simulink model "KD_cl_harness_cl_ouports_added"  (R2015b)
settings: Solver=ode45  StartTime=0  StopTime=inf  FixedStep=0.01  MaxStep=0.005  RelTol=1e-5  AbsTol=1e-5
undefined symbols (not defined in the file or in its folder): A2, bin_vec, c_0, c_1000, c_1000inv, c_100inv, c_1d2p4, c_1p7, c_4400inv, c_5500inv, c_80, c_compmap, c_ctok, c_fflow_max, c_fflow_min, c_filt, c_flowdiv, c_flowmin, c_flowmult, c_inf, c_km1d2k, c_n1, c_p00001, c_p01, c_p1e9, c_p4d1p4, c_pincomp, c_rair, c_roacorr, c_rpmtoradpers, c_svrthrottle1, c_svrthrottle2, c_svrthrottlearg, c_svrthrottlebeta, c_vnliftmax, c_vnliftmin, cl_offset, clff, Coefs, const, const_exhat, const_vec, Dual_array, dual_zero, egr_ecu_ff, expcon, f_mat, gs_jul, HQP_eps, HQP_INF, HQP_saturation, IV, L2, length_L, maxL, mHQP_saturation, minL, Newton, nRed, num_constraints ... (+22)
libraries: simulink x33
(part 4 of 6)

== system KD_cl_harness_cl_ouports_added/ctrl_rb_explicit_20140220_v6_simp/scheduled_observer/observer ==
  map : Inport
  egrr : Inport  Port=2
  xhatROpm : Inport  Port=3
  u : Inport  Port=4  OutDataTypeStr=single
  Action Port : ActionPort  ActionType=then
  Gain : Gain  Gain=expcon.RobsC  Multiplication=Matrix(K*u) (u vector)
      settings: AttributesFormatString=%<Multiplication>
  Gain1 : Gain  Gain=expcon.RobsL  Multiplication=Matrix(K*u) (u vector)
      settings: AttributesFormatString=%<Multiplication>
  Gain2 : Gain  Gain=expcon.RobsA  Multiplication=Matrix(K*u) (u vector)
      settings: AttributesFormatString=%<Multiplication>
  Gain3 : Gain  Gain=expcon.RobsB  Multiplication=Matrix(K*u) (u vector)
      settings: AttributesFormatString=%<Multiplication>
  Gain4 : Gain  Gain=expcon.RobsD  Multiplication=Matrix(K*u) (u vector)
      settings: AttributesFormatString=%<Multiplication>
  Mux : Mux  Inputs=2
  Mux1 : Mux  Inputs=3
  Sum : Sum  Inputs=++|
  Sum1 : Sum  Inputs=|+-
  Sum2 : Sum  Inputs=|++
  Sum3 : Sum  Inputs=+-|
  Sum4 : Sum  Inputs=-+|
  Sum5 : Sum  Inputs=+-|
  Unit Delay{1..4,7..8} (6 alike) : UnitDelay  SampleTime=-1
      settings: AttributesFormatString=%<X0>
  xhatRO : Outport  OutDataTypeStr=single
  xhat : Outport  Port=2  InitialOutput=[0,0,0,0,0,0]
  wires:
  Sum5/1 -> Mux/2
  Unit Delay4/1 -> Sum5/2
  Sum3/1 -> Mux/1
  Unit Delay3/1 -> Sum3/2
  Unit Delay1/1 -> Mux1/2
  Unit Delay2/1 -> Mux1/3
  [map] -> Unit Delay1/1
  [egrr] -> Unit Delay2/1
  Mux1/1 -> xhat/1
  Gain/1 -> Sum1/2
  Sum4/1 -> Sum1/1
  Gain3/1 -> Sum2/2
  Sum/1 -> Sum2/1
  xhatROpm/1 -> Unit Delay7/1
  map/1 -> Sum3/1, Unit Delay3/1, [map]
  egrr/1 -> Sum5/1, Unit Delay4/1, [egrr]
  Sum1/1 -> Gain1/1
  Gain1/1 -> Sum/1
  Gain2/1 -> Sum/2
  u/1 -> Unit Delay8/1
  Mux/1 -> Sum4/2
  Gain4/1 -> Sum4/1
  Sum2/1 -> Mux1/1, xhatRO/1
  Unit Delay8/1 -> Gain3/1, Gain4/1
  Unit Delay7/1 -> Gain/1, Gain2/1

== system KD_cl_harness_cl_ouports_added/ctrl_rb_explicit_20140220_v6_simp/set_point_maps/EGR_rate_map ==
  fuel_rate_mm3perst : Inport
  engine_speed : Inport  Port=2
  egr_ecu : Lookup2D  RowIndex=egr_ecu_ff.x  ColumnIndex=egr_ecu_ff.y  Table=egr_ecu_ff.z  LookUpMeth=Interpolation-Use End Values
      settings: AttributesFormatString=%<LookUpMeth>\n%<RowIndex>\n%<ColumnIndex>\n%<Table>
  EGR_rate_ref : Outport
  wires:
  egr_ecu/1 -> EGR_rate_ref/1
  fuel_rate_mm3perst/1 -> egr_ecu/2
  engine_speed/1 -> egr_ecu/1

== system KD_cl_harness_cl_ouports_added/ctrl_rb_explicit_20140220_v6_simp/set_point_maps/intake_pressure_map ==
  fuel_rate_mm3perst : Inport
  engine_speed : Inport  Port=2
  boost_pressure_map : Subsystem
  intake_manifold_pressure_ref : Outport
  wires:
  engine_speed/1 -> boost_pressure_map/2(engine_speed)
  fuel_rate_mm3perst/1 -> boost_pressure_map/1(fuel_rate_mm3perst)
  boost_pressure_map/1(intake_manifold_pressure) -> intake_manifold_pressure_ref/1

== system KD_cl_harness_cl_ouports_added/pre-throttle manifold/p_preThrottle/Cus_integrator ==
  in : Inport
  p_prethrottle (kPa)1 : Integrator  InitialCondition=IV.p_prethrottle  UpperSaturationLimit=maxL.p_PreThrottle  LowerSaturationLimit=minL.p_PreThrottle
  p_preThrottle : Outport
  wires:
  p_prethrottle (kPa)1/1 -> p_preThrottle/1
  in/1 -> p_prethrottle (kPa)1/1

== system KD_cl_harness_cl_ouports_added/EGR Throttle/EGR Throttle/Throttle Model2/Air Model_map_use ==
  TA[deg] : Inport
  Ne[rpm] : Inport  Port=2
  Pim[Pa] : Inport  Port=3
  Tim[K] : Inport  Port=4
  Pa[Pa] : Inport  Port=5
  Ta[K] : Inport  Port=6
  R_im : Inport  Port=7
  R_a : Inport  Port=8
  Back-Flow : Subsystem
  Forward-Flow : Subsystem
  Gain : Gain  Gain=-1
  Product : Product  Inputs=/*  SaturateOnIntegerOverflow=on  RndMeth=Zero  InputSameDT=on  OutDataTypeStr=Inherit: Same as first input
  Product1 : Product  Inputs=*//  SaturateOnIntegerOverflow=on  RndMeth=Zero  InputSameDT=on  OutDataTypeStr=Inherit: Same as first input
  Product3 : Product  Inputs=*//  SaturateOnIntegerOverflow=on  RndMeth=Zero  InputSameDT=on  OutDataTypeStr=Inherit: Same as first input
  Switch : Switch  Threshold=1  SaturateOnIntegerOverflow=on  InputSameDT=on
  mt[kg/sec] : Outport
  forwardmt : Outport  Port=2
  backwardmt : Outport  Port=3
  sat_out-37 : Outport  Port=4
  sat_out-38 : Outport  Port=5
  sat_out-39 : Outport  Port=6
  sat_out-40 : Outport  Port=7
  out-1 : Outport  Port=8
  out-3 : Outport  Port=9
  out-4 : Outport  Port=10
  wires:
  Product1/1 -> Forward-Flow/1(Ro_a)
  Switch/1 -> mt[kg/sec]/1
  Product/1 -> Switch/2, out-1/1
  TA[deg]/1 -> Forward-Flow/2(TA[deg]), Back-Flow/1(TA[deg])
  [Pa] -> Product/2, Forward-Flow/4(Pa), Back-Flow/4(Pa)
  Pim[Pa]/1 -> Forward-Flow/5(Pm), Product/1, Back-Flow/5(Pm), Product3/1
  Pa[Pa]/1 -> [Pa]
  Ta[K]/1 -> [Ta]
  R_a/1 -> [Ra]
  R_im/1 -> [Rim]
  [Ra] -> Product1/3
  [Pa] -> Product1/1
  [Ta] -> Product1/2
  [Rim] -> Product3/3
  Tim[K]/1 -> Product3/2
  Forward-Flow/1(mt_dot[kg/s]) -> Switch/1, forwardmt/1
  Product3/1 -> Back-Flow/3(Ro_m)
  Back-Flow/1(mt_dot[kg/s]) -> Gain/1
  Ne[rpm]/1 -> Forward-Flow/3(Ne[rpm]), Back-Flow/2(Ne[rpm])
  Gain/1 -> Switch/3, backwardmt/1
  Back-Flow/2(sat_out-37) -> sat_out-37/1
  Back-Flow/3(sat_out-38) -> sat_out-38/1
  Forward-Flow/2(sat_out-39) -> sat_out-39/1
  Forward-Flow/3(sat_out-40) -> sat_out-40/1
  Back-Flow/4(out-3) -> out-3/1
  Forward-Flow/4(out-4) -> out-4/1

== system KD_cl_harness_cl_ouports_added/EGR Valve/SVR EGR/EGR_model/Air Model_map_use ==
  TA[deg] : Inport
  Ne[rpm] : Inport  Port=2
  Pim[Pa] : Inport  Port=3
  Tim[K] : Inport  Port=4
  Pa[Pa] : Inport  Port=5
  Ta[K] : Inport  Port=6
  R_im : Inport  Port=7
  R_a : Inport  Port=8
  Back-Flow : Subsystem
  Forward-Flow : Subsystem
  Gain : Gain  Gain=-1
  Product : Product  Inputs=/*  SaturateOnIntegerOverflow=on  RndMeth=Zero  InputSameDT=on  OutDataTypeStr=Inherit: Same as first input
  Product1 : Product  Inputs=*//  SaturateOnIntegerOverflow=on  RndMeth=Zero  InputSameDT=on  OutDataTypeStr=Inherit: Same as first input
  Product3 : Product  Inputs=*//  SaturateOnIntegerOverflow=on  RndMeth=Zero  InputSameDT=on  OutDataTypeStr=Inherit: Same as first input
  Switch : Switch  Threshold=1  SaturateOnIntegerOverflow=on  InputSameDT=on
  mt[kg/sec] : Outport
  forwardmt : Outport  Port=2
  sat_out-41 : Outport  Port=3
  sat_out-42 : Outport  Port=4
  sat_out-43 : Outport  Port=5
  sat_out-44 : Outport  Port=6
  out-2 : Outport  Port=7
  out-5 : Outport  Port=8
  out-6 : Outport  Port=9
  wires:
  Ne[rpm]/1 -> Back-Flow/2(Ne[rpm]), Forward-Flow/3(Ne[rpm])
  Back-Flow/1(mt_dot[kg/s]) -> Gain/1  "rv"
  Product3/1 -> Back-Flow/3(Ro_m)
  Forward-Flow/1(mt_dot[kg/s]) -> forwardmt/1, Switch/1  "ff"
  Tim[K]/1 -> Product3/2
  [Rim] -> Product3/3
  [Ta] -> Product1/2
  [Pa] -> Product1/1
  [Ra] -> Product1/3
  R_im/1 -> [Rim]
  R_a/1 -> [Ra]
  Ta[K]/1 -> [Ta]
  Pa[Pa]/1 -> [Pa]
  Pim[Pa]/1 -> Product3/1, Back-Flow/5(Pm), Product/1, Forward-Flow/5(Pm)
  [Pa] -> Back-Flow/4(Pa), Forward-Flow/4(Pa), Product/2
  TA[deg]/1 -> Back-Flow/1(TA[deg]), Forward-Flow/2(TA[deg])
  Product/1 -> Switch/2, out-2/1  "pr_exhaust_by_intake"
  Switch/1 -> mt[kg/sec]/1
  Product1/1 -> Forward-Flow/1(Ro_a)
  Gain/1 -> Switch/3
  Back-Flow/2(sat_out-41) -> sat_out-41/1
  Back-Flow/3(sat_out-42) -> sat_out-42/1
  Forward-Flow/2(sat_out-43) -> sat_out-43/1
  Forward-Flow/3(sat_out-44) -> sat_out-44/1
  Back-Flow/4(out-5) -> out-5/1
  Forward-Flow/4(out-6) -> out-6/1

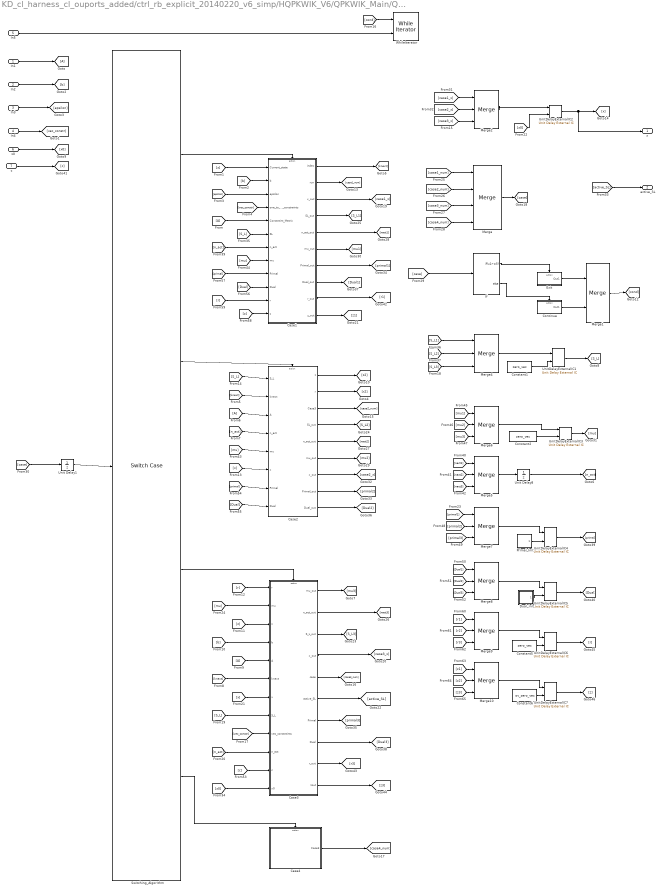
== system KD_cl_harness_cl_ouports_added/ctrl_rb_explicit_20140220_v6_simp/HQPKWIK_V6/QPKWIK_Main/QPKWIK_While_Loop ==
  In1 : Inport
  In2 : Inport  Port=2
  In3 : Inport  Port=3
  In4 : Inport  Port=4
  In5 : Inport  Port=5
  x0 : Inport  Port=6
  c : Inport  Port=7
  Case1 : Subsystem  TreatAsAtomicUnit=on
  Case2 : Subsystem  TreatAsAtomicUnit=on
  Case3 : Subsystem  TreatAsAtomicUnit=on
  Case4 : Subsystem  TreatAsAtomicUnit=on
  Constant1 : Constant  Value=zero_vec  VectorParams1D=off  OutDataTypeStr=int32
      settings: AttributesFormatString=%<Value>\n%<VectorParams1D>
  Constant2 : Constant  Value=zero_vec  VectorParams1D=off  OutDataTypeStr=single
      settings: AttributesFormatString=%<Value>\n%<VectorParams1D>
  Constant5 : Constant  Value=zero_vec  VectorParams1D=off  OutDataTypeStr=single
      settings: AttributesFormatString=%<Value>\n%<VectorParams1D>
  Constant6 : Constant  Value=ov_zero_vec  VectorParams1D=off  OutDataTypeStr=single
      settings: AttributesFormatString=%<Value>\n%<VectorParams1D>
  Continue : Subsystem  TreatAsAtomicUnit=on
  Dual_init : Subsystem
  Exit : Subsystem  TreatAsAtomicUnit=on
  If : If  IfExpression=u1>=5
  Merge : Merge  Inputs=4
  Merge1 : Merge  InitialOutput=1
      settings: AttributesFormatString=%<InitialOutput>
  Merge10 : Merge  Inputs=3  InitialOutput=ov_zero_vec
      settings: AttributesFormatString=%<InitialOutput>
  Merge2 : Merge  Inputs=3  InitialOutput=ov_zero_vec
      settings: AttributesFormatString=%<InitialOutput>
  Merge4 : Merge  Inputs=3  InitialOutput=zero_vec
      settings: AttributesFormatString=%<InitialOutput>
  Merge5 : Merge  Inputs=3  InitialOutput=0
      settings: AttributesFormatString=%<InitialOutput>
  Merge6 : Merge  Inputs=3  InitialOutput=zero_vec
      settings: AttributesFormatString=%<InitialOutput>
  Merge7 : Merge  Inputs=3  InitialOutput=primal_init
      settings: AttributesFormatString=%<InitialOutput>
  Merge8 : Merge  Inputs=3  InitialOutput=dual_zero
      settings: AttributesFormatString=%<InitialOutput>
  Merge9 : Merge  Inputs=3  InitialOutput=zero_vec
      settings: AttributesFormatString=%<InitialOutput>
  Primal_Init : Subsystem
  Switching_Algorithm : SwitchCase  CaseConditions={1,2,3}
  Unit Delay1 : UnitDelay  InitialCondition=1  SampleTime=-1
      settings: AttributesFormatString=%<X0>
  Unit Delay8 : UnitDelay  SampleTime=-1
      settings: AttributesFormatString=%<X0>
  UnitDelayExternalIC{1..7} (7 alike) : simulink/Additional Math & Discrete/Additional Discrete/Unit Delay External IC  tsamp=-1
  WhileIterator : WhileIterator  MaxIters=2000  ResetStates=reset
  x : Outport  InitialOutput=ov_zero_vec
  active_SL : Outport  Port=2
  wires:
  [x0] -> Case3/12(x0)
  [active_SL] -> active_SL/1
  Unit Delay1/1 -> Switching_Algorithm/1
  [z] -> Case1/12(z)
  [case] -> Unit Delay1/1
  Constant6/1 -> UnitDelayExternalIC7/2
  UnitDelayExternalIC7/1 -> [z]
  Merge10/1 -> UnitDelayExternalIC7/1
  [z1] -> Merge10/1
  [z2] -> Merge10/2
  [z3] -> Merge10/3
  Constant5/1 -> UnitDelayExternalIC6/2
  UnitDelayExternalIC6/1 -> [r]
  Merge9/1 -> UnitDelayExternalIC6/1
  [r1] -> Merge9/1
  [r2] -> Merge9/2
  [r3] -> Merge9/3
  [r] -> Case1/11(r)
  Case3/10(zout) -> [z3]
  Case3/9(r_out) -> [r3]
  Case1/10(z_out) -> [z1]
  Case1/9(r_out) -> [r1]
  Case2/4(SL_out) -> [S_L2]
  Case2/9(Dual_out) -> [Dual2]
  Case2/8(Primal_out) -> [primal2]
  Case1/8(Dual_out) -> [Dual1]
  Case1/7(Primal_out) -> [primal1]
  [Dual] -> Case1/10(Dual)
  [primal] -> Case1/9(Primal)
  [Dual] -> Case2/8(Dual)
  [primal] -> Case2/7(Primal)
  [c] -> Case3/11(c)
  c/1 -> [c]
  Case3/8(Dual) -> [Dual3]
  Case3/7(Primal) -> [primal3]
  Dual_init/1(Dual_init) -> UnitDelayExternalIC5/2
  UnitDelayExternalIC5/1 -> [Dual]
  Merge8/1 -> UnitDelayExternalIC5/1
  [Dual1] -> Merge8/1
  [Dual2] -> Merge8/2
  [Dual3] -> Merge8/3
  Primal_Init/1(Primal_init) -> UnitDelayExternalIC4/2
  UnitDelayExternalIC4/1 -> [primal]
  Merge7/1 -> UnitDelayExternalIC4/1
  [primal1] -> Merge7/1
  [primal2] -> Merge7/2
  [primal3] -> Merge7/3
  x0/1 -> [x0]
  [x0] -> UnitDelayExternalIC2/2
  [S_L] -> Case3/8(S_L)
  [n_act] -> Case2/4(n_act)
  Merge2/1 -> UnitDelayExternalIC2/1
  UnitDelayExternalIC2/1 -> x/1, [x]
  [S_L] -> Case2/1(S_L)
  [x] -> Case3/7(x)
  Unit Delay8/1 -> [n_act]
  [x] -> Case1/1(Current_state)
  [n_act] -> Case3/10(n_act)
  Case1/1(index) -> [knext]
  Exit/1(Out1) -> Merge1/1
  Continue/1(Out1) -> Merge1/2
  If/2 -> Continue/Action
  If/1 -> Exit/Action
  In5/1 -> WhileIterator/2
  Switching_Algorithm/4 -> Case4/Action
  [A] -> Case3/5(A)
  [knext] -> Case3/6(knext)
  [b] -> Case3/4(b)
  Case2/2(r) -> [r2]
  Case2/1(z) -> [z2]
  [knext] -> Case2/2(knext)
  [A] -> Case2/3(A)
  In4/1 -> [vec_constr]
  [z] -> Case3/3(z)
  [vec_constr] -> Case3/9(vec_constraints)
  [r] -> Case3/1(r)
  [vec_constr] -> Case1/4(one_to_numb_constraints)
  [epsilon] -> Case1/3(epsilon)
  [b] -> Case1/2(b)
  [A] -> Case1/5(Constraint_Matrix)
  In3/1 -> [epsilon]
  In2/1 -> [b]
  In1/1 -> [A]
  Switching_Algorithm/1 -> Case1/Action
  Case1/2(run) -> [case1_num]
  [case1_num] -> Merge/1
  Case2/3(Case3) -> [case2_num]
  [case2_num] -> Merge/2
  Case3/5(case) -> [case3_num]
  [case3_num] -> Merge/3
  Case4/1(Case3) -> [case4_num]
  [case4_num] -> Merge/4
  Merge/1 -> [case]
  [case] -> If/1
  Case1/3(x_out) -> [case1_x]
  [case1_x] -> Merge2/1
  Case3/4(x_out) -> [case3_x]
  [case2_x] -> Merge2/2
  Merge1/1 -> [cond]
  [cond] -> WhileIterator/1
  Switching_Algorithm/2 -> Case2/Action
  Case3/6(active_SL) -> [active_SL]
  Case1/4(SL_out) -> [S_L1]
  [S_L1] -> Merge4/1
  [S_L2] -> Merge4/2
  Case2/5(n_act_out) -> [nact2]
  Case3/3(S_L_out) -> [S_L3]
  Merge5/1 -> Unit Delay8/1
  Case3/2(n_act_out) -> [nact3]
  [nact1] -> Merge5/1
  [nact2] -> Merge5/2
  [nact3] -> Merge5/3
  [n_act] -> Case1/7(n_act)
  Case1/5(n_act_out) -> [nact1]
  Merge6/1 -> UnitDelayExternalIC3/1
  Constant2/1 -> UnitDelayExternalIC3/2
  [mu] -> Case3/2(mu)
  Case3/1(mu_out) -> [mu3]
  [mu] -> Case1/8(mu)
  [mu] -> Case2/5(mu)
  Case2/6(mu_out) -> [mu2]
  [mu1] -> Merge6/1
  [mu2] -> Merge6/2
  UnitDelayExternalIC3/1 -> [mu]
  Case1/6(mu_out) -> [mu1]
  Switching_Algorithm/3 -> Case3/Action
  [mu3] -> Merge6/3
  [x] -> Case2/6(x)
  Case2/7(x_out) -> [case2_x]
  [S_L] -> Case1/6(SL)
  Constant1/1 -> UnitDelayExternalIC1/2
  UnitDelayExternalIC1/1 -> [S_L]
  [case3_x] -> Merge2/3
  [S_L3] -> Merge4/3
  Merge4/1 -> UnitDelayExternalIC1/1

== system KD_cl_harness_cl_ouports_added/ctrl_rb_explicit_20140220_v6_simp/ntremap/remap_wt_to_map/ThrottleModel1 ==
  TA_deg : Inport
  Ne_rpm : Inport  Port=2
  Pim_Pa : Inport  Port=3
  Tamb_K : Inport  Port=4
  wegrthr : Inport  Port=5
  AirModel_map_use : Subsystem
  Ra : Constant  Value=c_rair  OutDataTypeStr=single  SampleTime=-1
      settings: AttributesFormatString=%<Value>\n%<SampleTime>
  p_pre_throttle : Outport  OutDataTypeStr=single
  sat_out-45 : Outport  Port=2
  sat_out-46 : Outport  Port=3
  sat_out-58 : Outport  Port=4
  sat_out-59 : Outport  Port=5
  sat_out-60 : Outport  Port=6
  sat_out-61 : Outport  Port=7
  sat_out-62 : Outport  Port=8
  sat_out-63 : Outport  Port=9
  sat_out-64 : Outport  Port=10
  sat_out-65 : Outport  Port=11
  out-17 : Outport  Port=12
  out-28 : Outport  Port=13
  wires:
  AirModel_map_use/1(p_pre_throttle) -> p_pre_throttle/1
  wegrthr/1 -> AirModel_map_use/6(wegrthr)
  Ne_rpm/1 -> AirModel_map_use/2(Ne_rpm)
  Ra/1 -> AirModel_map_use/5(R_a)
  Pim_Pa/1 -> AirModel_map_use/3(Pim_Pa)
  Tamb_K/1 -> AirModel_map_use/4(Ta_K)
  TA_deg/1 -> AirModel_map_use/1(TA_deg)
  AirModel_map_use/2(sat_out-45) -> sat_out-45/1
  AirModel_map_use/3(sat_out-46) -> sat_out-46/1
  AirModel_map_use/4(sat_out-58) -> sat_out-58/1
  AirModel_map_use/5(sat_out-59) -> sat_out-59/1
  AirModel_map_use/6(sat_out-60) -> sat_out-60/1
  AirModel_map_use/7(sat_out-61) -> sat_out-61/1
  AirModel_map_use/8(sat_out-62) -> sat_out-62/1
  AirModel_map_use/9(sat_out-63) -> sat_out-63/1
  AirModel_map_use/10(sat_out-64) -> sat_out-64/1
  AirModel_map_use/11(sat_out-65) -> sat_out-65/1
  AirModel_map_use/12(out-17) -> out-17/1
  AirModel_map_use/13(out-28) -> out-28/1

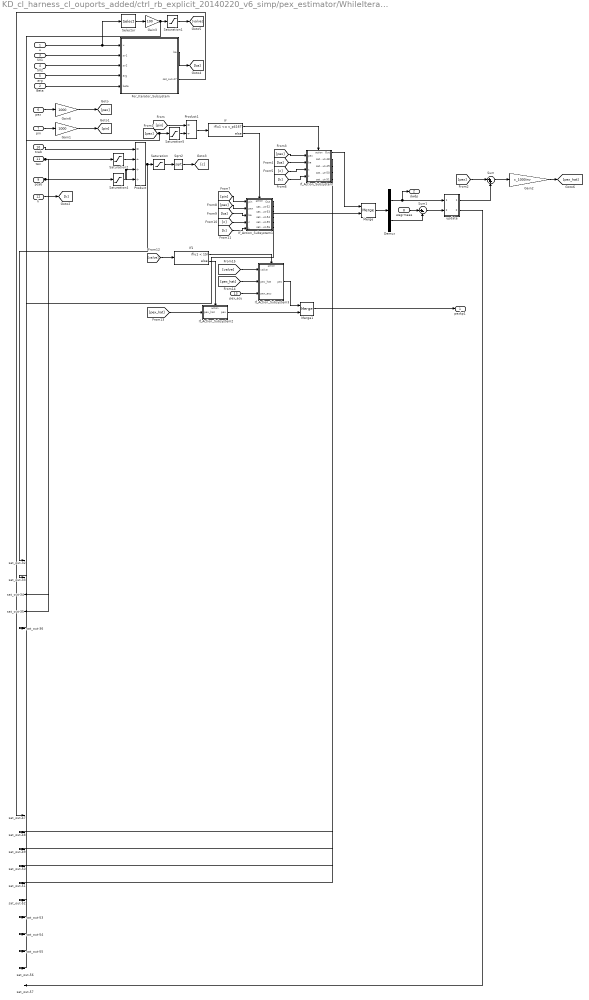
== system KD_cl_harness_cl_ouports_added/ctrl_rb_explicit_20140220_v6_simp/pex_estimator/WhileIteratorSubsystem/newton ==
  u : Inport
  Beta : Inport  Port=2
  SV1 : Inport  Port=3
  SV2 : Inport  Port=4
  arg : Inport  Port=5
  pex : Inport  Port=6
  pin : Inport  Port=7
  wegrmeas : Inport  Port=8
  pcab : Inport  Port=9
  tcab : Inport  Port=10
  tex : Inport  Port=11
  k : Inport  Port=12
  pex_ecu : Inport  Port=13
  Demux : Demux  Outputs=2
  For_Iterator_Subsystem : Subsystem  TreatAsAtomicUnit=on
  Gain1 : Gain  Gain=1000
      settings: AttributesFormatString=%<Gain>
  Gain2 : Gain  Gain=c_1000inv
      settings: AttributesFormatString=%<Gain>
  Gain3 : Gain  Gain=100
      settings: AttributesFormatString=%<Gain>
  Gain6 : Gain  Gain=1000
      settings: AttributesFormatString=%<Gain>
  If : If  IfExpression=u1 <= c_p4167
  If1 : If  IfExpression=u1 < 15
  If_Action_Subsystem : Subsystem  TreatAsAtomicUnit=on
  If_Action_Subsystem1 : Subsystem  TreatAsAtomicUnit=on
  If_Action_Subsystem2 : Subsystem  TreatAsAtomicUnit=on
  If_Action_Subsystem3 : Subsystem  TreatAsAtomicUnit=on
  Merge : Merge
  Merge1 : Merge
  Product : Product  Inputs=*///  RndMeth=Zero
  Product1 : Product  Inputs=*/  RndMeth=Zero
  Saturation : Saturate  UpperLimit=inf  LowerLimit=0
      settings: AttributesFormatString=%<LowerLimit>\n%<UpperLimit>
  Saturation1 : Saturate  UpperLimit=c_inf  LowerLimit=c_0
      settings: AttributesFormatString=%<LowerLimit>\n%<UpperLimit>
  Saturation2 : Saturate  UpperLimit=c_inf  LowerLimit=c_p1e9
      settings: AttributesFormatString=%<LowerLimit>\n%<UpperLimit>
  Saturation4 : Saturate  UpperLimit=c_inf  LowerLimit=c_p1e9
      settings: AttributesFormatString=%<LowerLimit>\n%<UpperLimit>
  Saturation5 : Saturate  UpperLimit=c_inf  LowerLimit=c_p1e9
      settings: AttributesFormatString=%<LowerLimit>\n%<UpperLimit>
  Selector : Selector  InputPortWidth=2  IndexOptions=Index vector (dialog)  Indices=1  OutputSizes=1
  Sqrt2 : Sqrt  AlgorithmType=Newton-Raphson  SaturateOnIntegerOverflow=on
  Sum : Sum  Inputs=|++
  Sum1 : Sum  Inputs=|+-
  update : Subsystem
  pexkp1 : Outport
  dwdp : Outport  Port=2
  sat_out-32 : Outport  Port=3
  sat_out-33 : Outport  Port=4
  sat_out-34 : Outport  Port=5
  sat_out-35 : Outport  Port=6
  sat_out-36 : Outport  Port=7
  sat_out-47 : Outport  Port=8
  sat_out-48 : Outport  Port=9
  sat_out-49 : Outport  Port=10
  sat_out-50 : Outport  Port=11
  sat_out-51 : Outport  Port=12
  sat_out-52 : Outport  Port=13
  sat_out-53 : Outport  Port=14
  sat_out-54 : Outport  Port=15
  sat_out-55 : Outport  Port=16
  sat_out-56 : Outport  Port=17
  sat_out-57 : Outport  Port=18
  wires:
  Saturation5/1 -> Product1/2
  Saturation4/1 -> Product/4, Product/3
  Saturation2/1 -> Product/2
  Saturation/1 -> Sqrt2/1
  Sum/1 -> Gain2/1
  update/1(delta) -> Sum/2
  [pex] -> Sum/1
  Merge/1 -> Demux/1
  If_Action_Subsystem1/1(Out) -> Merge/2
  If_Action_Subsystem/1(Out) -> Merge/1
  [k] -> If_Action_Subsystem1/5(k)
  [c] -> If_Action_Subsystem1/4(c)
  [ba] -> If_Action_Subsystem1/3(ba)
  [pex] -> If_Action_Subsystem1/2(pex)
  [pin] -> If_Action_Subsystem1/1(pin)
  If/2 -> If_Action_Subsystem1/Action
  [k] -> If_Action_Subsystem/4(k)
  [c] -> If_Action_Subsystem/3(c)
  [ba] -> If_Action_Subsystem/2(ba)
  [pex] -> If_Action_Subsystem/1(pex)
  If/1 -> If_Action_Subsystem/Action
  Product1/1 -> If/1
  [pex] -> Saturation5/1, sat_out-36/1
  [pin] -> Product1/1
  For_Iterator_Subsystem/1(ba) -> [ba]
  Product/1 -> Saturation/1, sat_out-32/1
  Gain1/1 -> [pin]
  Gain6/1 -> [pex]
  SV2/1 -> For_Iterator_Subsystem/3(sv2)
  k/1 -> [k]
  tex/1 -> Saturation2/1, sat_out-34/1
  tcab/1 -> Product/1
  pcab/1 -> Saturation4/1, sat_out-35/1
  wegrmeas/1 -> Sum1/1
  pin/1 -> Gain1/1
  pex/1 -> Gain6/1
  arg/1 -> For_Iterator_Subsystem/4(arg)
  SV1/1 -> For_Iterator_Subsystem/2(sv1)
  Beta/1 -> For_Iterator_Subsystem/5(beta)
  u/1 -> For_Iterator_Subsystem/1(u), Selector/1
  Demux/1 -> dwdp/1, update/1(dwdp)
  Demux/2 -> Sum1/2
  Sqrt2/1 -> [c]
  Selector/1 -> Gain3/1
  Gain3/1 -> Saturation1/1, sat_out-33/1
  Saturation1/1 -> [valve]
  [valve] -> If1/1
  If1/2 -> If_Action_Subsystem2/Action
  If1/1 -> If_Action_Subsystem3/Action
  Gain2/1 -> [pex_hat]
  [pex_hat] -> If_Action_Subsystem2/1(pex_hat)
  [valve] -> If_Action_Subsystem3/1(valve)
  [pex_hat] -> If_Action_Subsystem3/2(pex_hat)
  pex_ecu/1 -> If_Action_Subsystem3/3(pex_ecu)
  If_Action_Subsystem2/1(pex) -> Merge1/2
  If_Action_Subsystem3/1(pex) -> Merge1/1
  Merge1/1 -> pexkp1/1
  Sum1/1 -> update/2(error)
  For_Iterator_Subsystem/2(sat_out-47) -> sat_out-47/1
  If_Action_Subsystem/2(sat_out-48) -> sat_out-48/1
  If_Action_Subsystem/3(sat_out-49) -> sat_out-49/1
  If_Action_Subsystem/4(sat_out-50) -> sat_out-50/1
  If_Action_Subsystem/5(sat_out-51) -> sat_out-51/1
  If_Action_Subsystem1/2(sat_out-52) -> sat_out-52/1
  If_Action_Subsystem1/3(sat_out-53) -> sat_out-53/1
  If_Action_Subsystem1/4(sat_out-54) -> sat_out-54/1
  If_Action_Subsystem1/5(sat_out-55) -> sat_out-55/1
  If_Action_Subsystem1/6(sat_out-56) -> sat_out-56/1
  update/2(sat_out-57) -> sat_out-57/1

== system KD_cl_harness_cl_ouports_added/ctrl_rb_explicit_20140220_v6_simp/set_point_maps/intake_pressure_map/boost_pressure_map ==
  fuel_rate_mm3perst : Inport
  engine_speed : Inport  Port=2
  pim : Lookup2D  RowIndex=pim_ff.x  ColumnIndex=pim_ff.y  Table=pim_ff.z  LookUpMeth=Interpolation-Use End Values
      settings: AttributesFormatString=%<LookUpMeth>\n%<RowIndex>\n%<ColumnIndex>\n%<Table>
  intake_manifold_pressure : Outport
  wires:
  pim/1 -> intake_manifold_pressure/1
  fuel_rate_mm3perst/1 -> pim/2
  engine_speed/1 -> pim/1

== system KD_cl_harness_cl_ouports_added/EGR Throttle/EGR Throttle/Throttle Model2/Air Model_map_use/Back-Flow ==
  TA[deg] : Inport
  Ne[rpm] : Inport  Port=2
  Ro_m : Inport  Port=3
  Pa : Inport  Port=4
  Pm : Inport  Port=5
  Cal phi1 : Subsystem
  Constant1 : Constant  Value=(const.k/(2*(const.k+1)))^0.5
  Constant2 : Constant  Value=SVR_throttle.Beta
  Constant6 : Constant  Value=SVR_throttle.num_SV
  Constant7 : Constant  Value=SVR_throttle.SV
  Constant8 : Constant  Value=SVR_throttle.arg
  Gain : Gain  Gain=1/100
  Gain1 : Gain  Gain=1/5500
  Mux : Mux  Inputs=2
  Phi1 : Fcn  Expr=sqrt(((const.k-1)/(2*const.k)*(1-u)+u)*(1-u))
  Pm-Pa1 : Product  Inputs=/*  SaturateOnIntegerOverflow=on  RndMeth=Zero  InputSameDT=on  OutDataTypeStr=Inherit: Same as first input
  SVR_throttle : MATLAB Function  TreatAsAtomicUnit=on
  Saturation : Saturate  UpperLimit=inf  LowerLimit=0
  Saturation1 : Saturate  UpperLimit=1.0  LowerLimit=1/(const.k+1)
  Switch1 : Switch  Criteria=u2 > Threshold  Threshold=1/(const.k+1)
  correct flow2 : Product  Inputs=***  SaturateOnIntegerOverflow=on  RndMeth=Zero  InputSameDT=on  OutDataTypeStr=Inherit: Same as first input
  tokgps1 : Gain  Gain=1/1000
  mt_dot[kg/s] : Outport
  sat_out-37 : Outport  Port=2
  sat_out-38 : Outport  Port=3
  out-3 : Outport  Port=4
  wires:
  Cal phi1/1(phi) -> correct flow2/1
  Constant1/1 -> Switch1/3
  Switch1/1 -> correct flow2/3
  Saturation1/1 -> Phi1/1
  Phi1/1 -> Switch1/1
  correct flow2/1 -> tokgps1/1
  tokgps1/1 -> mt_dot[kg/s]/1
  Pm-Pa1/1 -> Switch1/2, Saturation1/1, sat_out-38/1, out-3/1
  Pm/1 -> Pm-Pa1/1, Cal phi1/1(Pm)
  Pa/1 -> Pm-Pa1/2
  Ro_m/1 -> Cal phi1/2(Ro_m)
  SVR_throttle/1(B_A_spd) -> Saturation/1, sat_out-37/1
  TA[deg]/1 -> Gain/1
  Gain/1 -> Mux/1
  Gain1/1 -> Mux/2
  Ne[rpm]/1 -> Gain1/1
  Constant6/1 -> SVR_throttle/2(num_SV)
  Constant2/1 -> SVR_throttle/3(Beta)
  Constant7/1 -> SVR_throttle/4(SV)
  Constant8/1 -> SVR_throttle/5(arg)
  Mux/1 -> SVR_throttle/1(u)
  Saturation/1 -> correct flow2/2

== system KD_cl_harness_cl_ouports_added/EGR Throttle/EGR Throttle/Throttle Model2/Air Model_map_use/Forward-Flow ==
  Ro_a : Inport
  TA[deg] : Inport  Port=2
  Ne[rpm] : Inport  Port=3
  Pa : Inport  Port=4
  Pm : Inport  Port=5
  Cal phi : Subsystem
  Constant1 : Constant  Value=(const.k/(2*(const.k+1)))^0.5
  Constant2 : Constant  Value=SVR_throttle.Beta
  Constant6 : Constant  Value=SVR_throttle.num_SV
  Constant7 : Constant  Value=SVR_throttle.SV
  Constant8 : Constant  Value=SVR_throttle.arg
  Gain : Gain  Gain=1/100
  Gain1 : Gain  Gain=1/5500
  Mux : Mux  Inputs=2
  Phi1 : Fcn  Expr=sqrt(((const.k-1)/(2*const.k)*(1-u)+u)*(1-u))
  Pm-Pa1 : Product  Inputs=*/  SaturateOnIntegerOverflow=on  RndMeth=Zero  InputSameDT=on  OutDataTypeStr=Inherit: Same as first input
  SVR_throttle : MATLAB Function  TreatAsAtomicUnit=on
  Saturation : Saturate  UpperLimit=inf  LowerLimit=0
  Saturation1 : Saturate  UpperLimit=1.0  LowerLimit=1/(const.k+1)
  Switch1 : Switch  Criteria=u2 > Threshold  Threshold=1/(const.k+1)
  correct flow2 : Product  Inputs=***  SaturateOnIntegerOverflow=on  RndMeth=Zero  InputSameDT=on  OutDataTypeStr=Inherit: Same as first input
  tokgps1 : Gain  Gain=1/1000
  mt_dot[kg/s] : Outport
  sat_out-39 : Outport  Port=2
  sat_out-40 : Outport  Port=3
  out-4 : Outport  Port=4
  wires:
  Cal phi/1(phi) -> correct flow2/1
  Constant1/1 -> Switch1/3
  Switch1/1 -> correct flow2/3
  Saturation1/1 -> Phi1/1
  Phi1/1 -> Switch1/1
  correct flow2/1 -> tokgps1/1
  tokgps1/1 -> mt_dot[kg/s]/1
  Pm-Pa1/1 -> Switch1/2, Saturation1/1, sat_out-40/1, out-4/1
  Pm/1 -> Pm-Pa1/1
  Pa/1 -> Pm-Pa1/2, Cal phi/1(Pa)
  Ro_a/1 -> Cal phi/2(Ro_a)
  Mux/1 -> SVR_throttle/1(u)
  TA[deg]/1 -> Gain/1
  Gain/1 -> Mux/1
  Gain1/1 -> Mux/2
  Ne[rpm]/1 -> Gain1/1
  SVR_throttle/1(B_A_spd) -> Saturation/1, sat_out-39/1
  Constant6/1 -> SVR_throttle/2(num_SV)
  Constant2/1 -> SVR_throttle/3(Beta)
  Constant7/1 -> SVR_throttle/4(SV)
  Constant8/1 -> SVR_throttle/5(arg)
  Saturation/1 -> correct flow2/2  "B(TA)(g/s)"

== system KD_cl_harness_cl_ouports_added/EGR Valve/SVR EGR/EGR_model/Air Model_map_use/Back-Flow ==
  TA[deg] : Inport
  Ne[rpm] : Inport  Port=2
  Ro_m : Inport  Port=3
  Pa : Inport  Port=4
  Pm : Inport  Port=5
  Cal phi1 : Subsystem
  Constant1 : Constant  Value=(const.k/(2*(const.k+1)))^0.5
  Constant2 : Constant  Value=SVR_EGR.Beta
  Constant6 : Constant  Value=SVR_EGR.num_SV
  Constant7 : Constant  Value=SVR_EGR.SV
  Constant8 : Constant  Value=SVR_EGR.arg
  Gain : Gain  Gain=1/100
  Gain1 : Gain  Gain=1/5500
  Gain2 : Gain  Gain=1/1000
  Mux : Mux  Inputs=2
  Phi1 : Fcn  Expr=sqrt(((const.k-1)/(2*const.k)*(1-u)+u)*(1-u))
  Pm-Pa1 : Product  Inputs=/*  SaturateOnIntegerOverflow=on  RndMeth=Zero  InputSameDT=on  OutDataTypeStr=Inherit: Same as first input
  SVR_EGR : MATLAB Function  TreatAsAtomicUnit=on
  Saturation : Saturate  UpperLimit=inf  LowerLimit=0
  Saturation1 : Saturate  UpperLimit=1.0  LowerLimit=1/(const.k+1)
  Switch1 : Switch  Criteria=u2 > Threshold  Threshold=1/(const.k+1)
  correct flow2 : Product  Inputs=***  SaturateOnIntegerOverflow=on  RndMeth=Zero  InputSameDT=on  OutDataTypeStr=Inherit: Same as first input
  mt_dot[kg/s] : Outport
  sat_out-41 : Outport  Port=2
  sat_out-42 : Outport  Port=3
  out-5 : Outport  Port=4
  wires:
  Gain2/1 -> mt_dot[kg/s]/1
  Mux/1 -> SVR_EGR/1(u)
  Constant8/1 -> SVR_EGR/5(arg)
  Constant7/1 -> SVR_EGR/4(SV)
  Constant2/1 -> SVR_EGR/3(Beta)
  Constant6/1 -> SVR_EGR/2(num_SV)
  Ne[rpm]/1 -> Gain1/1
  Gain1/1 -> Mux/2
  Gain/1 -> Mux/1
  TA[deg]/1 -> Gain/1
  SVR_EGR/1(B_A_spd) -> Saturation/1, sat_out-41/1
  Ro_m/1 -> Cal phi1/2(Ro_m)
  Pa/1 -> Pm-Pa1/2
  Pm/1 -> Cal phi1/1(Pm), Pm-Pa1/1
  Pm-Pa1/1 -> Saturation1/1, Switch1/2, sat_out-42/1, out-5/1
  correct flow2/1 -> Gain2/1
  Phi1/1 -> Switch1/1
  Saturation1/1 -> Phi1/1
  Switch1/1 -> correct flow2/3
  Constant1/1 -> Switch1/3
  Cal phi1/1(phi) -> correct flow2/1
  Saturation/1 -> correct flow2/2

== system KD_cl_harness_cl_ouports_added/EGR Valve/SVR EGR/EGR_model/Air Model_map_use/Forward-Flow ==
  Ro_a : Inport
  TA[deg] : Inport  Port=2
  Ne[rpm] : Inport  Port=3
  Pa : Inport  Port=4
  Pm : Inport  Port=5
  Cal phi : Subsystem
  Constant1 : Constant  Value=(const.k/(2*(const.k+1)))^0.5
  Constant3 : Constant  Value=SVR_EGR.Beta
  Constant4 : Constant  Value=SVR_EGR.num_SV
  Constant5 : Constant  Value=SVR_EGR.SV
  Constant9 : Constant  Value=SVR_EGR.arg
  Gain : Gain  Gain=1/100
  Gain1 : Gain  Gain=1/4400
  Gain2 : Gain  Gain=1/1000
  Mux : Mux  Inputs=2
  Phi1 : Fcn  Expr=sqrt(((const.k-1)/(2*const.k)*(1-u)+u)*(1-u))
  Pm-Pa1 : Product  Inputs=*/  SaturateOnIntegerOverflow=on  RndMeth=Zero  InputSameDT=on  OutDataTypeStr=Inherit: Same as first input
  SVR_EGR : MATLAB Function  TreatAsAtomicUnit=on
  Saturation : Saturate  UpperLimit=inf  LowerLimit=0
  Saturation1 : Saturate  UpperLimit=1.0  LowerLimit=1/(const.k+1)
  Switch1 : Switch  Criteria=u2 > Threshold  Threshold=1/(const.k+1)
  correct flow2 : Product  Inputs=***  SaturateOnIntegerOverflow=on  RndMeth=Zero  InputSameDT=on  OutDataTypeStr=Inherit: Same as first input
  mt_dot[kg/s] : Outport
  sat_out-43 : Outport  Port=2
  sat_out-44 : Outport  Port=3
  out-6 : Outport  Port=4
  wires:
  Gain2/1 -> mt_dot[kg/s]/1
  Constant9/1 -> SVR_EGR/5(arg)
  Constant5/1 -> SVR_EGR/4(SV)
  Constant3/1 -> SVR_EGR/3(Beta)
  Constant4/1 -> SVR_EGR/2(num_SV)
  SVR_EGR/1(B_A_spd) -> Saturation/1, sat_out-43/1
  Ne[rpm]/1 -> Gain1/1
  Gain1/1 -> Mux/2
  Gain/1 -> Mux/1
  TA[deg]/1 -> Gain/1
  Mux/1 -> SVR_EGR/1(u)
  Ro_a/1 -> Cal phi/2(Ro_a)
  Pa/1 -> Cal phi/1(Pa), Pm-Pa1/2
  Pm/1 -> Pm-Pa1/1
  Pm-Pa1/1 -> Saturation1/1, Switch1/2, sat_out-44/1, out-6/1
  correct flow2/1 -> Gain2/1
  Phi1/1 -> Switch1/1
  Saturation1/1 -> Phi1/1
  Switch1/1 -> correct flow2/3
  Constant1/1 -> Switch1/3
  Cal phi/1(phi) -> correct flow2/1
  Saturation/1 -> correct flow2/2  "B(TA)(g/s)"

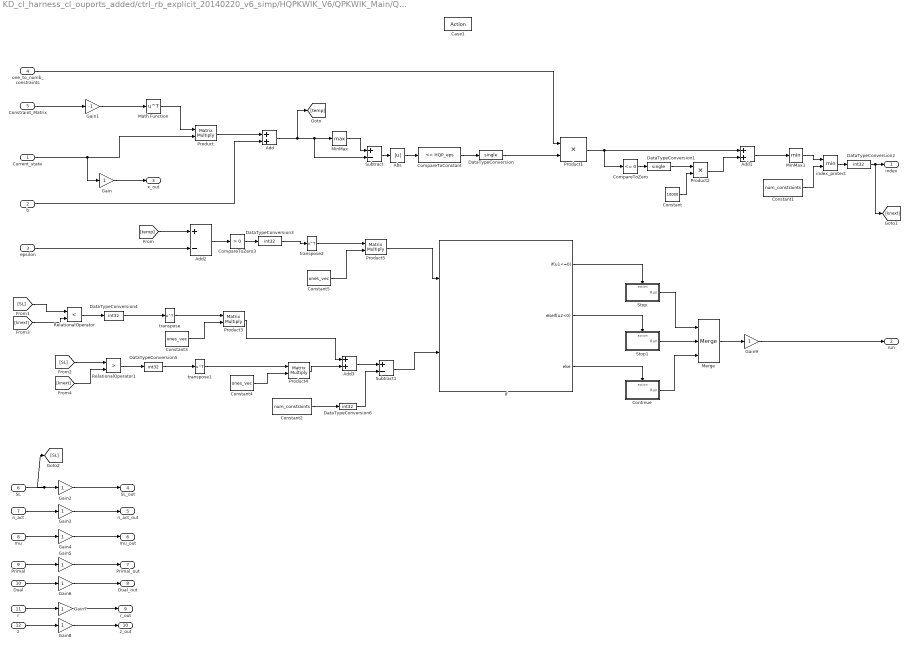
== system KD_cl_harness_cl_ouports_added/ctrl_rb_explicit_20140220_v6_simp/HQPKWIK_V6/QPKWIK_Main/QPKWIK_While_Loop/Case1 ==
  Current_state : Inport
  b : Inport  Port=2
  epsilon : Inport  Port=3
  one_to_numb_constraints : Inport  Port=4
  Constraint_Matrix : Inport  Port=5
  SL : Inport  Port=6
  n_act : Inport  Port=7
  mu : Inport  Port=8
  Primal : Inport  Port=9
  Dual : Inport  Port=10
  r : Inport  Port=11
  z : Inport  Port=12
  Case1 : ActionPort  ActionType=case
  Abs : Abs
  Add : Sum
  Add1 : Sum
  Add2 : Sum  Inputs=+-
  Add3 : Sum  OutDataTypeStr=int32
  CompareToConstant : simulink/Logic and Bit Operations/Compare To Constant  relop=<=  const=HQP_eps  OutDataTypeStr=boolean
  CompareToZero : simulink/Logic and Bit Operations/Compare To Zero  relop=<=  OutDataTypeStr=boolean
  CompareToZero3 : simulink/Logic and Bit Operations/Compare To Zero  relop=>  OutDataTypeStr=boolean
  Constant : Constant  Value=10000  OutDataTypeStr=single
  Constant1 : Constant  Value=num_constraints  OutDataTypeStr=single
  Constant2 : Constant  Value=num_constraints  OutDataTypeStr=double
  Constant3 : Constant  Value=ones_vec  VectorParams1D=off  OutDataTypeStr=int32
      settings: AttributesFormatString=%<VectorParams1D>
  Constant4 : Constant  Value=ones_vec  VectorParams1D=off  OutDataTypeStr=int32
      settings: AttributesFormatString=%<VectorParams1D>
  Constant5 : Constant  Value=ones_vec  VectorParams1D=off  OutDataTypeStr=int32
      settings: AttributesFormatString=%<VectorParams1D>
  Continue : Subsystem  TreatAsAtomicUnit=on
  DataTypeConversion : DataTypeConversion  OutDataTypeStr=single
  DataTypeConversion1 : DataTypeConversion  OutDataTypeStr=single
  DataTypeConversion{2..6} (5 alike) : DataTypeConversion  OutDataTypeStr=int32
  Gain{,4..8} (6 alike) : Gain
  Gain1 : Gain  Gain=-1
  Gain2 : Gain  OutDataTypeStr=int32
  Gain3 : Gain  OutDataTypeStr=int32
  Gain9 : Gain  OutDataTypeStr=uint8
  If : If  NumInputs=2  IfExpression=u1<=0  ElseIfExpressions=u2<0
  Math Function : Math  Operator=transpose  SaturateOnIntegerOverflow=on
  Merge : Merge  Inputs=3
  MinMax : MinMax  Function=max
      settings: AttributesFormatString=%<Function>
  MinMax1 : MinMax  OutDataTypeStr=single
  Product : Product  Multiplication=Matrix(*)  RndMeth=Zero
  Product1 : Product  RndMeth=Zero
  Product2 : Product  RndMeth=Zero
  Product3 : Product  Multiplication=Matrix(*)  OutDataTypeStr=int32  RndMeth=Zero
  Product4 : Product  Multiplication=Matrix(*)  OutDataTypeStr=int32  RndMeth=Zero
  Product5 : Product  Multiplication=Matrix(*)  OutDataTypeStr=int32  RndMeth=Zero
  RelationalOperator : RelationalOperator  Operator=<  OutDataTypeStr=boolean
  RelationalOperator1 : RelationalOperator  Operator=>  OutDataTypeStr=boolean
  Stop : Subsystem  TreatAsAtomicUnit=on
  Stop1 : Subsystem  TreatAsAtomicUnit=on
  Subtract : Sum  Inputs=+-
  Subtract1 : Sum  Inputs=+-  OutDataTypeStr=int32
  index_protect : MinMax  Inputs=2
  transpose : Math  Operator=transpose  SaturateOnIntegerOverflow=on
  transpose1 : Math  Operator=transpose  SaturateOnIntegerOverflow=on
  transpose2 : Math  Operator=transpose  SaturateOnIntegerOverflow=on
  index : Outport  InitialOutput=1
  run : Outport  Port=2  InitialOutput=2
  x_out : Outport  Port=3  InitialOutput=ov_zero_vec
  SL_out : Outport  Port=4  InitialOutput=zero_vec
  n_act_out : Outport  Port=5  InitialOutput=0
  mu_out : Outport  Port=6  InitialOutput=zero_vec
  Primal_out : Outport  Port=7  InitialOutput=primal_init
  Dual_out : Outport  Port=8  InitialOutput=dual_zero
  r_out : Outport  Port=9  InitialOutput=zero_vec
  z_out : Outport  Port=10  InitialOutput=ov_zero_vec
  wires:
  DataTypeConversion5/1 -> transpose1/1
  DataTypeConversion2/1 -> index/1, [knext]
  DataTypeConversion6/1 -> Subtract1/2
  DataTypeConversion4/1 -> transpose/1
  DataTypeConversion3/1 -> transpose2/1
  DataTypeConversion1/1 -> Product2/1
  DataTypeConversion/1 -> Product1/2
  Continue/1(Run) -> Merge/3
  Stop1/1(Run) -> Merge/2
  If/2 -> Stop1/Action
  Subtract1/1 -> If/2
  Constant2/1 -> DataTypeConversion6/1
  Add3/1 -> Subtract1/1
  If/3 -> Continue/Action
  Product4/1 -> Add3/2
  RelationalOperator1/1 -> DataTypeConversion5/1
  RelationalOperator/1 -> DataTypeConversion4/1
  [knext] -> RelationalOperator1/2
  [knext] -> RelationalOperator/2
  [SL] -> RelationalOperator1/1
  [SL] -> RelationalOperator/1
  z/1 -> Gain8/1
  Gain8/1 -> z_out/1
  r/1 -> Gain7/1
  Gain7/1 -> r_out/1
  Gain6/1 -> Dual_out/1
  Dual/1 -> Gain6/1
  Gain5/1 -> Primal_out/1
  Primal/1 -> Gain5/1
  one_to_numb_constraints/1 -> Product1/1
  MinMax/1 -> Subtract/1
  Merge/1 -> Gain9/1
  CompareToZero3/1 -> DataTypeConversion3/1
  Stop/1(Run) -> Merge/1
  If/1 -> Stop/Action
  Product5/1 -> If/1
  Add2/1 -> CompareToZero3/1
  [temp] -> Add2/1
  epsilon/1 -> Add2/2
  b/1 -> Add/2
  Product/1 -> Add/1
  Current_state/1 -> Gain/1, Product/2
  Math Function/1 -> Product/1
  Constraint_Matrix/1 -> Gain1/1
  Gain1/1 -> Math Function/1
  Product1/1 -> Add1/1, CompareToZero/1
  Add1/1 -> MinMax1/1
  CompareToZero/1 -> DataTypeConversion1/1
  Constant/1 -> Product2/2
  Product2/1 -> Add1/2
  Add/1 -> MinMax/1, Subtract/2, [temp]
  Gain/1 -> x_out/1
  MinMax1/1 -> index_protect/1
  index_protect/1 -> DataTypeConversion2/1
  Constant1/1 -> index_protect/2
  Subtract/1 -> Abs/1
  Abs/1 -> CompareToConstant/1
  CompareToConstant/1 -> DataTypeConversion/1
  SL/1 -> [SL], Gain2/1
  Gain2/1 -> SL_out/1
  n_act/1 -> Gain3/1
  Gain3/1 -> n_act_out/1
  mu/1 -> Gain4/1
  Gain4/1 -> mu_out/1
  Gain9/1 -> run/1
  transpose/1 -> Product3/1
  Product3/1 -> Add3/1
  Constant3/1 -> Product3/2
  transpose1/1 -> Product4/1
  Constant4/1 -> Product4/2
  transpose2/1 -> Product5/1
  Constant5/1 -> Product5/2

== system KD_cl_harness_cl_ouports_added/ctrl_rb_explicit_20140220_v6_simp/HQPKWIK_V6/QPKWIK_Main/QPKWIK_While_Loop/Case2 ==
  S_L : Inport
  knext : Inport  Port=2
  A : Inport  Port=3
  n_act : Inport  Port=4  OutDataTypeStr=int32
  mu : Inport  Port=5
  x : Inport  Port=6
  Primal : Inport  Port=7
  Dual : Inport  Port=8
  Case2 : ActionPort  ActionType=case
  Constant3 : Constant  Value=3  OutDataTypeStr=uint8
  Dual_direction : Subsystem  TreatAsAtomicUnit=on
  Gain : Gain  OutDataTypeStr=int32
  Gain1 : Gain  OutDataTypeStr=int32
  Gain{2..5} (4 alike) : Gain
  If : If
  Merge : Merge
  Nominal_dual_direction : Subsystem  TreatAsAtomicUnit=on
  Product : Product  Multiplication=Matrix(*)  RndMeth=Zero
  extracts_ith_page_of_array : Selector  NumberOfDimensions=2  IndexOptions=Select all,Index vector (port)  Indices=[1:3],[1:3]  OutputSizes=1,1
  z : Outport  InitialOutput=ov_zero_vec
  r : Outport  Port=2  InitialOutput=zero_vec
  Case3 : Outport  Port=3  InitialOutput=3
  SL_out : Outport  Port=4  InitialOutput=zero_vec
  n_act_out : Outport  Port=5  InitialOutput=0
  mu_out : Outport  Port=6  InitialOutput=zero_vec
  x_out : Outport  Port=7  InitialOutput=ov_zero_vec
  Primal_out : Outport  Port=8  InitialOutput=primal_init
  Dual_out : Outport  Port=9  InitialOutput=dual_zero
  wires:
  Primal/1 -> Gain5/1, Product/1
  Gain5/1 -> Primal_out/1
  Gain4/1 -> Dual_out/1
  Dual/1 -> Gain4/1, [Dual_arraycase2]
  [nactcase2] -> If/1
  Product/1 -> z/1
  Merge/1 -> r/1
  Nominal_dual_direction/1(r) -> Merge/2
  Dual_direction/1(r) -> Merge/1
  If/1 -> Dual_direction/Action
  Constant3/1 -> Case3/1
  S_L/1 -> Gain/1
  A/1 -> [Acase2]
  [Acase2] -> extracts_ith_page_of_array/1
  knext/1 -> [knextcase2]
  [knextcase2] -> extracts_ith_page_of_array/2
  n_act/1 -> [nactcase2], Gain1/1
  If/2 -> Nominal_dual_direction/Action
  extracts_ith_page_of_array/1 -> [Aknextcase2]
  [Aknextcase2] -> Product/2
  [Aknextcase2] -> Dual_direction/2(Aknext)
  [Dual_arraycase2] -> Dual_direction/1(Dual_array)
  Gain/1 -> SL_out/1
  Gain1/1 -> n_act_out/1
  mu/1 -> Gain2/1
  Gain2/1 -> mu_out/1
  Gain3/1 -> x_out/1
  x/1 -> Gain3/1

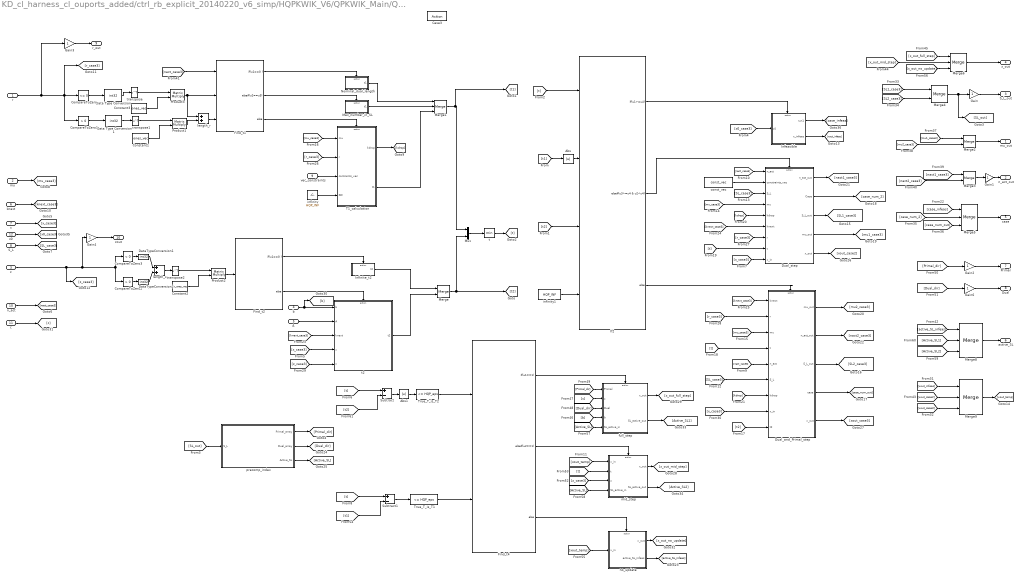
== system KD_cl_harness_cl_ouports_added/ctrl_rb_explicit_20140220_v6_simp/HQPKWIK_V6/QPKWIK_Main/QPKWIK_While_Loop/Case3 ==
  r : Inport
  mu : Inport  Port=2
  z : Inport  Port=3
  b : Inport  Port=4
  A : Inport  Port=5
  knext : Inport  Port=6
  x : Inport  Port=7
  S_L : Inport  Port=8
  vec_constraints : Inport  Port=9
  n_act : Inport  Port=10
  c : Inport  Port=11
  x0 : Inport  Port=12
  Case3 : ActionPort  ActionType=case
  Abs : Abs
  Abs1 : Abs
  CompareToZero : simulink/Logic and Bit Operations/Compare To Zero  relop=<=  OutDataTypeStr=boolean
  CompareToZero1 : simulink/Logic and Bit Operations/Compare To Zero  relop=>  OutDataTypeStr=boolean
  CompareToZero2 : simulink/Logic and Bit Operations/Compare To Zero  relop=>  OutDataTypeStr=boolean
  CompareToZero3 : simulink/Logic and Bit Operations/Compare To Zero  relop=<  OutDataTypeStr=boolean
  Constant1 : Constant  Value=ones_vec  VectorParams1D=off  OutDataTypeStr=int32
      settings: AttributesFormatString=%<VectorParams1D>
  Constant2 : Constant  Value=ov_ones_vec  VectorParams1D=off  OutDataTypeStr=int32
      settings: AttributesFormatString=%<VectorParams1D>
  Constant3 : Constant  Value=ones_vec  VectorParams1D=off  OutDataTypeStr=int32
      settings: AttributesFormatString=%<VectorParams1D>
  Data Type Conversion : DataTypeConversion  OutDataTypeStr=int32
  Data Type Conversion1 : DataTypeConversion  OutDataTypeStr=int32
  DataTypeConversion1 : DataTypeConversion  OutDataTypeStr=int32
  DataTypeConversion2 : DataTypeConversion  OutDataTypeStr=int32
  Dual_and_Primal_step : Subsystem  TreatAsAtomicUnit=on
  Dual_step : Subsystem  TreatAsAtomicUnit=on
  Find_t1 : If  NumInputs=3  IfExpression=u1==0  ElseIfExpressions=u2==u3
  Find_t2 : If  IfExpression=u1==0
  Find_t4 : If  NumInputs=2  IfExpression=u1==1  ElseIfExpressions=u2==1
  Gain : Gain  OutDataTypeStr=int32
  Gain1 : Gain  OutDataTypeStr=int32
  Gain{2..4,6} (4 alike) : Gain
  If2 : If  NumInputs=4  IfExpression=u1>=u4  ElseIfExpressions=u3>=u4 & u2<u4
  Infeasible : Subsystem  TreatAsAtomicUnit=on
  Infinite_t2 : Subsystem  TreatAsAtomicUnit=on
  Max_number_in_SL : Subsystem  TreatAsAtomicUnit=on
  Merge : Merge
  Merge{1,5..6,8..9} (5 alike) : Merge  Inputs=3
      Merge5 settings: AttributesFormatString=%<InitialOutput>
      Merge6 settings: AttributesFormatString=%<InitialOutput>
      Merge8 settings: AttributesFormatString=%<InitialOutput>
      Merge9 settings: AttributesFormatString=%<InitialOutput>
  Merge2 : Merge
      settings: AttributesFormatString=%<InitialOutput>
  Merge3 : Merge  InitialOutput=0
      settings: AttributesFormatString=%<InitialOutput>
  Merge4 : Merge  InitialOutput=zero_vec
      settings: AttributesFormatString=%<InitialOutput>
  Mux : Mux  Inputs=2
  Nominal_dual_length : Subsystem  TreatAsAtomicUnit=on
  Product1 : Product  Multiplication=Matrix(*)  OutDataTypeStr=int32  RndMeth=Zero
  Product2 : Product  Multiplication=Matrix(*)  OutDataTypeStr=int32  RndMeth=Zero
  Product3 : Product  Multiplication=Matrix(*)  OutDataTypeStr=int32  RndMeth=Zero
  Subtract : Sum  Inputs=+-
  Subtract1 : Sum  Inputs=+-
  T1_calculation : Subsystem  TreatAsAtomicUnit=on
  True_T_is_T1 : simulink/Logic and Bit Operations/Compare To Constant  relop=<=  const=HQP_eps  OutDataTypeStr=boolean
  True_T_is_T2 : simulink/Logic and Bit Operations/Compare To Constant  relop=<=  const=HQP_eps  OutDataTypeStr=boolean
  const_vec : Constant  Value=const_vec  VectorParams1D=off  OutDataTypeStr=single
      settings: AttributesFormatString=%<VectorParams1D>
  full_step : Subsystem  TreatAsAtomicUnit=on
  infinity : Constant  Value=HQP_INF  OutDataTypeStr=single
  infinity1 : Constant  Value=HQP_INF  OutDataTypeStr=single
  length_r : Sum
  length_z : Sum
  mid_step : Subsystem  TreatAsAtomicUnit=on
  no_update : Subsystem  TreatAsAtomicUnit=on
  precomp_index : Subsystem
  t : MinMax
  t2 : Subsystem  TreatAsAtomicUnit=on
  transpose : Math  Operator=transpose  SaturateOnIntegerOverflow=on
  transpose1 : Math  Operator=transpose  SaturateOnIntegerOverflow=on
  transpose2 : Math  Operator=transpose  SaturateOnIntegerOverflow=on
  mu_out : Outport  InitialOutput=zero_vec
  n_act_out : Outport  Port=2  OutDataTypeStr=int32  InitialOutput=0
  S_L_out : Outport  Port=3  InitialOutput=zero_vec
  x_out : Outport  Port=4  InitialOutput=ov_zero_vec
  case : Outport  Port=5  InitialOutput=2
  active_SL : Outport  Port=6  InitialOutput=0
  Primal : Outport  Port=7  InitialOutput=primal_init
  Dual : Outport  Port=8  InitialOutput=dual_zero
  r_out : Outport  Port=9  InitialOutput=zero_vec
  zout : Outport  Port=10  InitialOutput=ov_zero_vec
  wires:
  Abs1/1 -> True_T_is_T2/1
  True_T_is_T1/1 -> Find_t4/2
  Subtract1/1 -> True_T_is_T1/1
  [t1] -> Subtract1/2
  [t] -> Subtract1/1
  True_T_is_T2/1 -> Find_t4/1
  Subtract/1 -> Abs1/1
  [t2] -> Subtract/2
  [t] -> Subtract/1
  [t2] -> Dual_and_Primal_step/9(t2)
  DataTypeConversion2/1 -> length_z/2
  DataTypeConversion1/1 -> length_z/1
  x0/1 -> [x0_case3]
  [Active_SL2] -> Merge8/3
  Merge8/1 -> active_SL/1
  [active_SL_infeas] -> Merge8/1
  [Active_SL1] -> Merge8/2
  mid_step/2(SL_active_out) -> [Active_SL2]
  [Active_SL] -> mid_step/4(SL_active_in)
  full_step/2(SL_active_out) -> [Active_SL1]
  [Active_SL] -> full_step/5(SL_active_in)
  no_update/2(active_SL_infeas) -> [active_SL_infeas]
  Find_t4/3 -> no_update/Action
  Find_t4/2 -> mid_step/Action
  no_update/1(x_out) -> [x_out_no_update]
  [xout_temp] -> no_update/1(x_in)
  [z_case3] -> mid_step/3(z)
  [t] -> mid_step/2(t)
  Gain4/1 -> zout/1
  Gain3/1 -> r_out/1
  Gain2/1 -> Primal/1
  Gain6/1 -> Dual/1
  [Dual_dir] -> Gain6/1
  [Primal_dir] -> Gain2/1
  [Primal_dir] -> full_step/1(Primal)
  [Dual_dir] -> full_step/3(Dual)
  [c] -> full_step/2(c)
  [b] -> full_step/4(b)
  c/1 -> [c]
  full_step/1(x_out) -> [x_out_full_step]
  Find_t4/1 -> full_step/Action
  mid_step/1(x_out) -> [x_out_mid_step]
  [xout_temp] -> mid_step/1(x_in)
  Merge9/1 -> [xout_temp]
  [xout_case3] -> Merge9/3
  [xout_case2] -> Merge9/2
  [xout_infeas] -> Merge9/1
  Dual_and_Primal_step/5(x_out) -> [xout_case3]
  Dual_step/5(x_out) -> [xout_case2]
  [x_case3] -> Dual_and_Primal_step/8(x_in)
  [x_case3] -> Dual_step/9(x_in)
  precomp_index/3(Active_SL) -> [Active_SL]
  precomp_index/2(Dual_array) -> [Dual_dir]
  precomp_index/1(Primal_array) -> [Primal_dir]
  [SL_out] -> precomp_index/1(S_L)
  mu/1 -> [mu_case3]
  S_L/1 -> [SL_case3]
  [x_case3] -> t2/4(x)
  Merge4/1 -> [SL_out], Gain/1
  const_vec/1 -> Dual_step/2(constraints_vec)
  Product2/1 -> Find_t2/1
  infinity/1 -> T1_calculation/4(INF)
  vec_constraints/1 -> T1_calculation/3(contraints_vec)
  Merge5/1 -> case/1
  Merge3/1 -> Gain1/1
  Merge2/1 -> mu_out/1
  infinity1/1 -> If2/4
  t/1 -> [t]
  [t2] -> If2/3
  Abs/1 -> If2/2
  [t1] -> Abs/1
  Mux/1 -> t/1
  Merge1/1 -> Mux/1, [t1]
  Merge/1 -> Mux/2, [t2]
  t2/1(t2) -> Merge/2
  Infinite_t2/1(t2) -> Merge/1
  T1_calculation/2(t1) -> Merge1/3
  Nominal_dual_length/1(t1) -> Merge1/1
  Max_number_in_SL/1(t1) -> Merge1/2
  A/1 -> t2/2(A)
  b/1 -> [b], t2/1(b)
  Find_t2/2 -> t2/Action
  Find_t2/1 -> Infinite_t2/Action
  length_z/1 -> transpose2/1
  CompareToZero2/1 -> DataTypeConversion2/1
  CompareToZero3/1 -> DataTypeConversion1/1
  z/1 -> Gain4/1, CompareToZero2/1, CompareToZero3/1, [z_case3]
  Product1/1 -> length_r/2
  length_r/1 -> Find_t1/3
  CompareToZero1/1 -> Data Type Conversion1/1
  Product3/1 -> Find_t1/2, length_r/1
  CompareToZero/1 -> Data Type Conversion/1
  r/1 -> Gain3/1, CompareToZero/1, CompareToZero1/1, [r_case3]
  Find_t1/3 -> T1_calculation/Action
  Find_t1/2 -> Max_number_in_SL/Action
  Find_t1/1 -> Nominal_dual_length/Action
  [t] -> If2/1
  Infeasible/1(run1) -> [case_infeas]
  x/1 -> [x_case3]
  n_act/1 -> [nact_case3]
  [nact_case3] -> Dual_and_Primal_step/5(n_act)
  [SL_case3] -> Dual_and_Primal_step/6(S_L)
  [SL_case3] -> Dual_step/3(S_L)
  [mu_case3] -> Dual_step/4(mu)
  [mu_case3] -> Dual_and_Primal_step/3(mu)
  [mu_case3] -> T1_calculation/1(mu)
  [t] -> Dual_and_Primal_step/4(t)
  [t] -> Dual_step/8(t)
  T1_calculation/1(kdrop) -> [kdrop]
  [kdrop] -> Dual_and_Primal_step/7(kdrop)
  knext/1 -> [knext_case3]
  [knext_case3] -> t2/3(knext)
  [knext_case3] -> Dual_step/6(knext)
  [knext_case3] -> Dual_and_Primal_step/1(knext)
  [r_case3] -> Dual_step/7(r)
  [r_case3] -> Dual_and_Primal_step/2(r)
  [z_case3] -> t2/5(z)
  Infeasible/2(x_infeas) -> [xout_infeas]
  Dual_step/3(S_L_out) -> [SL1_case3]
  Dual_and_Primal_step/3(S_L_out) -> [SL2_case3]
  [SL1_case3] -> Merge4/1
  [SL2_case3] -> Merge4/2
  Dual_and_Primal_step/4(case) -> [case_num_out]
  Dual_step/2(Case) -> [case_num_2]
  Dual_step/4(mu_out) -> [mu1_case3]
  [mu1_case3] -> Merge2/1
  [mu2_case3] -> Merge2/2
  Dual_step/1(n_act_out) -> [nact1_case3]
  Dual_and_Primal_step/2(n_act_out) -> [nact2_case3]
  [nact2_case3] -> Merge3/2
  [nact1_case3] -> Merge3/1
  [nact_case3] -> Find_t1/1
  [r_case3] -> T1_calculation/2(r)
  [x0_case3] -> Infeasible/1(x0)
  [kdrop] -> Dual_step/5(kdrop)
  [nact_case3] -> Dual_step/1(n_act)
  Dual_and_Primal_step/1(mu_out) -> [mu2_case3]
  If2/3 -> Dual_and_Primal_step/Action
  If2/2 -> Dual_step/Action
  If2/1 -> Infeasible/Action
  Data Type Conversion/1 -> transpose/1
  Data Type Conversion1/1 -> transpose1/1
  Gain/1 -> S_L_out/1
  Gain1/1 -> n_act_out/1
  [x_out_no_update] -> Merge6/3
  [x_out_full_step] -> Merge6/1
  [x_out_mid_step] -> Merge6/2
  Merge6/1 -> x_out/1
  [case_infeas] -> Merge5/1
  [case_num_2] -> Merge5/2
  [case_num_out] -> Merge5/3
  transpose/1 -> Product3/1
  Constant3/1 -> Product3/2
  transpose1/1 -> Product1/1
  Constant1/1 -> Product1/2
  transpose2/1 -> Product2/1
  Constant2/1 -> Product2/2

== system KD_cl_harness_cl_ouports_added/ctrl_rb_explicit_20140220_v6_simp/HQPKWIK_V6/QPKWIK_Main/QPKWIK_While_Loop/Case4 ==
  Case4 : ActionPort  ActionType=default
  Exit_criteria : Constant  Value=5  OutDataTypeStr=uint8
  Case3 : Outport  InitialOutput=5
  wires:
  Exit_criteria/1 -> Case3/1

== system KD_cl_harness_cl_ouports_added/ctrl_rb_explicit_20140220_v6_simp/HQPKWIK_V6/QPKWIK_Main/QPKWIK_While_Loop/Continue ==
  Continue : ActionPort  ActionType=else
  True : Constant  OutDataTypeStr=boolean
  Out1 : Outport  InitialOutput=1
  wires:
  True/1 -> Out1/1

== system KD_cl_harness_cl_ouports_added/ctrl_rb_explicit_20140220_v6_simp/HQPKWIK_V6/QPKWIK_Main/QPKWIK_While_Loop/Dual_init ==
  Dual_Array : Constant  Value=Dual_array  OutDataTypeStr=single
  extracts_ith_page_of_array1 : Selector  NumberOfDimensions=3  IndexOptions=Select all,Select all,Index vector (port)  Indices=[1:10],[1:3],[1:3]  OutputSizes=1,1,1
  size_dual : Constant  Value=size_dual  OutDataTypeStr=single
  Dual_init : Outport
  wires:
  extracts_ith_page_of_array1/1 -> Dual_init/1
  size_dual/1 -> extracts_ith_page_of_array1/2
  Dual_Array/1 -> extracts_ith_page_of_array1/1

== system KD_cl_harness_cl_ouports_added/ctrl_rb_explicit_20140220_v6_simp/HQPKWIK_V6/QPKWIK_Main/QPKWIK_While_Loop/Exit ==
  Exit : ActionPort  ActionType=then
  False : Constant  Value=0  OutDataTypeStr=boolean
  Out1 : Outport  InitialOutput=0
  wires:
  False/1 -> Out1/1

== system KD_cl_harness_cl_ouports_added/ctrl_rb_explicit_20140220_v6_simp/HQPKWIK_V6/QPKWIK_Main/QPKWIK_While_Loop/Primal_Init ==
  Primal_Array : Constant  Value=Primal_array  OutDataTypeStr=single
  extracts_ith_page_of_array : Selector  NumberOfDimensions=3  IndexOptions=Select all,Select all,Index vector (port)  Indices=[1:3],[1:3],[1:3]  OutputSizes=1,1,1
  size_primal : Constant  Value=size_primal  OutDataTypeStr=single
  Primal_init : Outport
  wires:
  extracts_ith_page_of_array/1 -> Primal_init/1
  size_primal/1 -> extracts_ith_page_of_array/2
  Primal_Array/1 -> extracts_ith_page_of_array/1
